simulink model "IMU_MODEL"  (R2018b)
settings: Solver=VariableStepAuto  StartTime=0.0  StopTime=10.0  RelTol=1e-3
libraries: simulink x1
settings Model: Creator=Paweł Tymiński  LastModifiedBy=Paweł Tymiński
settings SFSimCC: SimUseLocalCustomCode=off
settings RTWCC: RTWUseLocalCustomCode=off
settings CodeAppCC: StateflowObjectComments=on

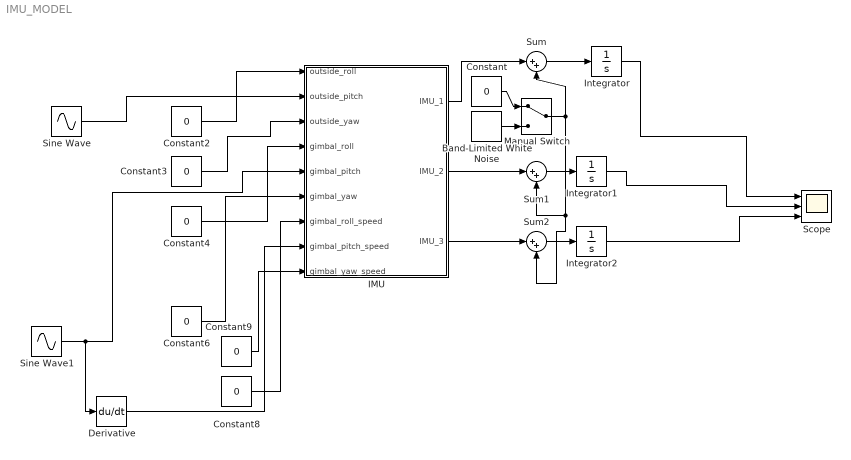
== system IMU_MODEL ==
  Band-Limited White Noise : simulink/Sources/Band-Limited White Noise  Cov=[0.1]  Ts=0.1  seed=[23341]
  Constant{,2..4,6,8..9} (7 alike) : Constant  Value=0
  Derivative : Derivative
  IMU : MATLAB Function  TreatAsAtomicUnit=on
  Integrator : Integrator
  Integrator1 : Integrator
  Integrator2 : Integrator
  Manual Switch : ManualSwitch
  Scope : Scope  NumInputPorts=3
  Sine Wave : Sin  Phase=pi/4  SampleTime=0
  Sine Wave1 : Sin  SampleTime=0
  Sum : Sum  Inputs=|++
  Sum1 : Sum  Inputs=|++
  Sum2 : Sum  Inputs=|++
  wires:
  Constant9/1 -> IMU/9(gimbal_yaw_speed)
  IMU/1(IMU_1) -> Sum/1
  Sine Wave/1 -> IMU/2(outside_pitch)
  Constant4/1 -> IMU/4(gimbal_roll)
  Constant6/1 -> IMU/6(gimbal_yaw)
  IMU/3(IMU_3) -> Sum2/1
  IMU/2(IMU_2) -> Sum1/1
  Integrator2/1 -> Scope/3
  Manual Switch/1 -> Sum2/2, Sum1/2, Sum/2
  Sum2/1 -> Integrator2/1
  Sum1/1 -> Integrator1/1
  Sum/1 -> Integrator/1
  Integrator1/1 -> Scope/2
  Integrator/1 -> Scope/1
  Band-Limited White Noise/1 -> Manual Switch/2
  Constant/1 -> Manual Switch/1
  Constant3/1 -> IMU/3(outside_yaw)
  Constant8/1 -> IMU/7(gimbal_roll_speed)
  Sine Wave1/1 -> Derivative/1, IMU/5(gimbal_pitch)
  Derivative/1 -> IMU/8(gimbal_pitch_speed)
  Constant2/1 -> IMU/1(outside_roll)

== matlab function IMU_MODEL/IMU ==
  data: outside_roll input; IMU_1 output; outside_pitch input; outside_yaw input; gimbal_roll input; gimbal_pitch input; gimbal_yaw input; gimbal_roll_speed input; gimbal_pitch_speed input; gimbal_yaw_speed input; IMU_2 output; IMU_3 output

function [IMU_1, IMU_2, IMU_3] = IMU(outside_roll,outside_pitch,outside_yaw,gimbal_roll , gimbal_pitch , gimbal_yaw , gimbal_roll_speed ,gimbal_pitch_speed , gimbal_yaw_speed )
% kąty gimbala
theta_1 = gimbal_yaw ;
theta_2 = gimbal_pitch ;
theta_3 = gimbal_roll ;

J_0 =[1 0 0;
    0 cos(theta_1) -sin(theta_1);
   -sin(theta_2) cos(theta_2)*sin(theta_1) cos(theta_1)*cos(theta_2)];
Phi_0 = [outside_yaw; outside_pitch; outside_roll];

Omega_phi = J_0*Phi_0;

Omega = [gimbal_yaw_speed; gimbal_pitch_speed; gimbal_roll_speed];

J = [cos(theta_2)*cos(theta_3) sin(theta_3) 0;
    cos(theta_2)*sin(theta_3) cos(theta_3) 0;
    -sin(theta_2) 0 1];
A=J*(Omega_phi + Omega);

IMU_1 = A(1); %yaw
IMU_2 = A(2); %pitch
IMU_3 = A(3); %roll

end
